simulink model "diffBlocks"  (R2023b)
settings: Solver=VariableStepAuto  StartTime=0.0  StopTime=10.0  RelTol=1e-3
libraries: visionanalysis x1, aerolibschedule x1
settings Model: Creator=neham  LastModifiedBy=neham

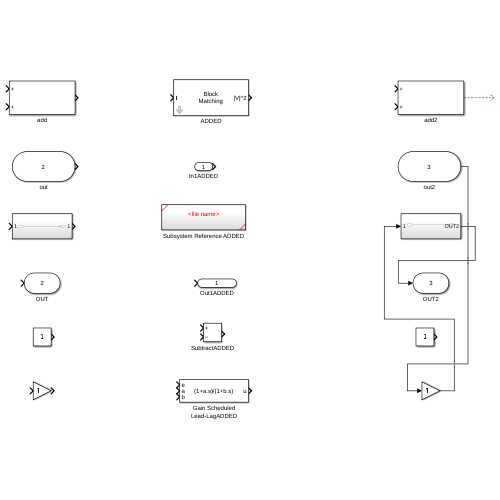
[thumbnail: Simulink's stored preview of the top-level diagram]
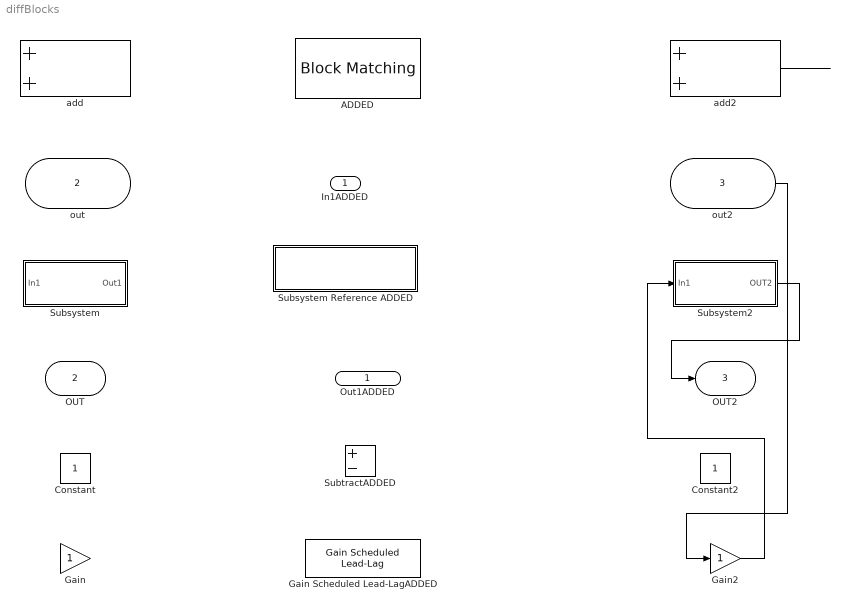
== system diffBlocks ==
  In1ADDED : Inport
  out : Inport  Port=2
  out2 : Inport  Port=3
  ADDED : visionanalysis/Block Matching  which2img=Current frame and N-th frame back  N=1  searchMethod=Exhaustive  matchCriteria=Mean square error (MSE)  blockSize=[17 17]  overlapping=[0 0]  maxDisplacement=[7 7]  outVelForm=Magnitude-squared  roundingMode=Floor  overflowMode=on  prodOutputMode=Binary point scaling  prodOutputWordLength=32  prodOutputFracLength=0  accumMode=Binary point scaling  accumWordLength=32  accumFracLength=0  outputMode=Binary point scaling  outputWordLength=8  outputFracLength=0
  Constant : Constant
  Constant2 : Constant
  Gain : Gain
  Gain Scheduled Lead-LagADDED : aerolibschedule/Gain Scheduled Lead-Lag  x_initial=0
  Gain2 : Gain
  Subsystem : Subsystem
  Subsystem Reference ADDED : Subsystem  ReferencedSubsystem=<file name>
  Subsystem2 : Subsystem
  SubtractADDED : Sum  Inputs=+-
  add : Sum
  add2 : Sum
  Out1ADDED : Outport  VectorParamsAs1DForOutWhenUnconnected=off
  OUT : Outport  Port=2
  OUT2 : Outport  Port=3
  wires:
  Subsystem2/1(OUT2) -> OUT2/1
  out2/1 -> Gain2/1
  Gain2/1 -> Subsystem2/1(In1)
  add2/1 -> ?

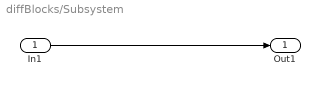
== system diffBlocks/Subsystem ==
  In1 : Inport
  Out1 : Outport
  wires:
  In1/1 -> Out1/1

== system diffBlocks/Subsystem Reference ADDED ==

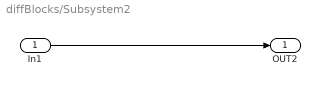
== system diffBlocks/Subsystem2 ==
  In1 : Inport
  OUT2 : Outport
  wires:
  In1/1 -> OUT2/1
